simulink model "Control_Schematic_13a"  (Simulink 8.3)
settings: Solver=ode3  StartTime=0.0  StopTime=350  FixedStep=Ts  RelTol=1e-3
values from neighbouring files (symbols this model uses):
  b = 156    [StartUp_1.m]    (also in StartUp_11_Validation.m; StartUp_3.m; StartUp_4.m; StartUp_7.m)
  Eps = .1    (= 0.1)    [StartUp_9.m]
  K1 = PolyCon(1,2)    [StartUp_1.m]    (also in StartUp_4.m = 1; StartUp_7.m = 16; StartUp_8.m = 16; StartUp_9.m = 0.23)
  k2 = floor(rk(2,1))    [StartUp_9.m]
  K2 = 2    [StartUp_4.m]    (also in StartUp_7.m = 8; StartUp_8.m = 8; StartUp_9.m = 0.83)
  K3 = 12000    [StartUp_9.m]
  Kn = .0019    (= 0.0019)    [StartUp_9.m]
  r = 820    [StartUp_1.m]    (also in StartUp_11_Validation.m = 50; StartUp_3.m = 520; StartUp_4.m = 0.01; StartUp_7.m = 0.01)
  TD = ss(Atd,Btd,Ctd,Dtd,Ts)    [StartUp_1.m]    (also in StartUp_3.m; StartUp_4.m; StartUp_7.m; StartUp_8.m)
  Ts = 1/1000    (= 0.001)    [StartUp_1.m]    (also in StartUp_11_Validation.m = 0.01; StartUp_3.m; StartUp_4.m; StartUp_7.m)
  x_0 = 2500    [StartUp_9.m]
  y_0 = 2500    [StartUp_9.m]
undefined symbols (not defined in the file or in its folder): d0t, DiscIntNeverNeededParam, dt, ht, k1, rho1, rho2, rt
libraries: simulink x2, dspinverses x1
settings Model: Creator=baqumau  LastModifiedBy=baqumau
settings DataIOCC: SignalLoggingSaveFormat=Dataset
settings DebuggingCC: UnderspecifiedInitializationDetection=Simplified  StateNameClashWarn=none
settings GRTTargetCC: CombineOutputUpdateFcns=on  GRTInterface=off

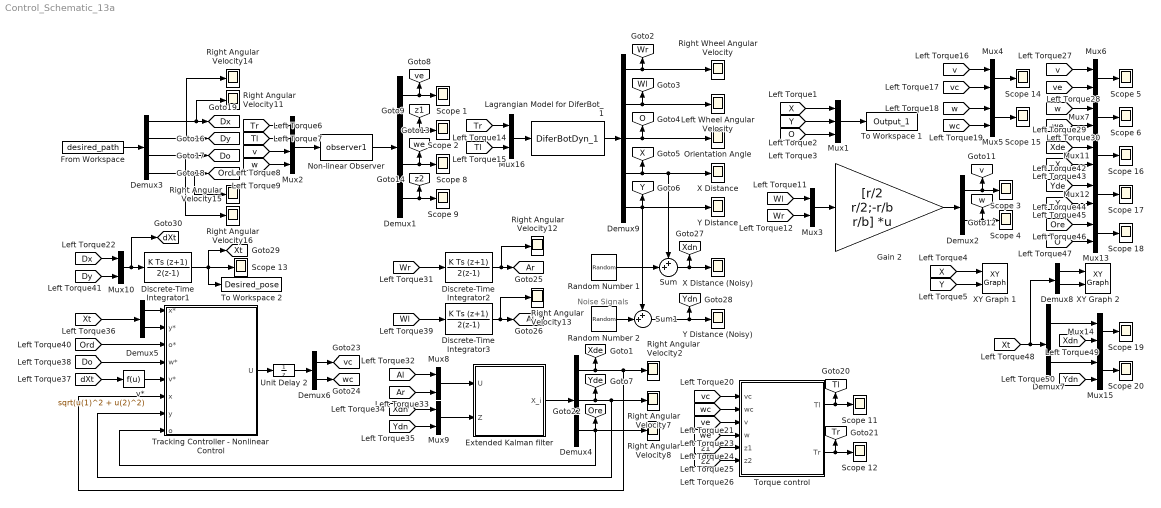
== system Control_Schematic_13a ==
  note: Noise Signals
  Demux1 : Demux
  Demux{2,5..8} (5 alike) : Demux  Outputs=2
  Demux3 : Demux
  Demux4 : Demux  Outputs=3
  Demux9 : Demux  Outputs=5
  Discrete-Time Integrator1 : DiscreteIntegrator  IntegratorMethod=Integration: Trapezoidal  gainval=1  InitialCondition=[x_0,y_0]'  SampleTime=Ts  ICPrevOutput=DiscIntNeverNeededParam  ICPrevScaledInput=DiscIntNeverNeededParam
  Discrete-Time Integrator2 : DiscreteIntegrator  IntegratorMethod=Integration: Trapezoidal  gainval=1  SampleTime=Ts  ICPrevOutput=DiscIntNeverNeededParam  ICPrevScaledInput=DiscIntNeverNeededParam
  Discrete-Time Integrator3 : DiscreteIntegrator  IntegratorMethod=Integration: Trapezoidal  gainval=1  SampleTime=Ts  ICPrevOutput=DiscIntNeverNeededParam  ICPrevScaledInput=DiscIntNeverNeededParam
  Extended Kalman filter : Subsystem
  From Workspace : FromWorkspace  VariableName=desired_path  SampleTime=Ts  OutputAfterFinalValue=Holding final value
  Gain 2 : Gain  Gain=[r/2 r/2;-r/b r/b]  Multiplication=Matrix(K*u)
  Lagrangian Model for DiferBot_1 : S-Function  FunctionName=DiferBotDyn_1  Parameters=par  EnableBusSupport=off
  Left Wheel Angular Velocity : Scope
      settings: YMin=-1  YMax=1  SaveName=ScopeData2
  Mux1 : Mux  Inputs=3
  Mux{3..16} (14 alike) : Mux  Inputs=2
  Mux2 : Mux
  Non-linear Observer : S-Function  FunctionName=observer1  Parameters=par  EnableBusSupport=off
  Orientation Angle : Scope
      settings: YMin=-3  YMax=3
  Random Number 1 : RandomNumber  Variance=.5  Seed=6  SampleTime=Ts
  Random Number 2 : RandomNumber  Variance=.5  Seed=8  SampleTime=Ts
  Right Angular Velocity{2,7..8,11..16} (9 alike) : Scope
      Right Angular Velocity11 settings: YMin=0  YMax=4500  SaveName=ScopeData17
      Right Angular Velocity12 settings: YMin=-3  YMax=30  SaveName=ScopeData39
      Right Angular Velocity13 settings: YMin=-3  YMax=3  SaveName=ScopeData40
      Right Angular Velocity14 settings: TimeRange=500  YMin=0  YMax=4500  SaveName=ScopeData20
      Right Angular Velocity15 settings: YMin=-3.141592653589793  YMax=3.141592653589793  SaveName=ScopeData15
      Right Angular Velocity16 settings: YMin=-0.1  YMax=-0.1  SaveName=ScopeData16
      Right Angular Velocity2 settings: YMin=2400  YMax=2600  SaveName=ScopeData35
      Right Angular Velocity7 settings: YMin=0  YMax=5000  SaveName=ScopeData36
      Right Angular Velocity8 settings: YMin=-3.141592653589793  YMax=3.141592653589793  SaveName=ScopeData37
  Right Wheel Angular Velocity : Scope
      settings: YMin=-1  YMax=20  SaveName=ScopeData3
  Scope {1..6,8..9,11..20} (18 alike) : Scope
      Scope 1 settings: YMin=0  YMax=5000  SaveName=ScopeData5
      Scope 11 settings: YMin=-20  YMax=20  SaveName=ScopeData24
      Scope 12 settings: YMin=-15  YMax=15  SaveName=ScopeData25
      Scope 13 settings: YMin=100  YMax=5000  SaveName=ScopeData42
      Scope 14 settings: YMin=-150  YMax=150  SaveName=ScopeData18
      Scope 15 settings: YMin=-2  YMax=2  SaveName=ScopeData19
      Scope 16 settings: YMin=0  YMax=5000  SaveName=ScopeData43
      Scope 17 settings: YMin=0  YMax=10000  SaveName=ScopeData46
      Scope 18 settings: YMin=-10  YMax=1.1  SaveName=ScopeData51
      Scope 19 settings: YMin=0  YMax=5000  SaveName=ScopeData52
      Scope 2 settings: YMin=-100  YMax=200  SaveName=ScopeData6
      Scope 20 settings: YMin=0  YMax=5000  SaveName=ScopeData53
      Scope 3 settings: YMin=0  YMax=5000  SaveName=ScopeData10
      Scope 4 settings: YMin=0  YMax=5000  SaveName=ScopeData11
      Scope 5 settings: YMin=-150  YMax=500  SaveName=ScopeData28
      Scope 6 settings: SaveName=ScopeData29
      Scope 8 settings: YMin=-1  YMax=1  SaveName=ScopeData12
      Scope 9 settings: TimeRange=388  YMin=-6  YMax=6  SaveName=ScopeData14
  Sum : Sum  Inputs=++|
  Sum1 : Sum  Inputs=++|
  To Workspace 1 : ToWorkspace  VariableName=Output_1  SaveFormat=Structure With Time  SampleTime=-1
  To Workspace 2 : ToWorkspace  VariableName=Desired_pose  SaveFormat=Structure With Time  SampleTime=-1
  Torque control : Subsystem
  Tracking Controller - Nonlinear Control : Subsystem
  Unit Delay 2 : UnitDelay  SampleTime=-1
  X Distance : Scope
      settings: YMin=0  YMax=5000  SaveName=ScopeData4
  X Distance (Noisy) : Scope
      settings: YMin=0  YMax=2600  SaveName=ScopeData38
  XY Graph 1 : simulink/Sinks/XY Graph  xmin=0  xmax=5000  ymin=0  ymax=5000  st=-1
  XY Graph 2 : simulink/Sinks/XY Graph  xmin=0  xmax=5000  ymin=0  ymax=5000  st=-1
  Y Distance : Scope
      settings: YMin=0  YMax=5000
  Y Distance (Noisy) : Scope
      settings: YMin=0  YMax=2600  SaveName=ScopeData41
  v* : Fcn  Expr=sqrt(u(1)^2 + u(2)^2)
  tag scope: Al=global, Ar=global, Do=global, Dx=global, Dy=global, O=global, Ord=global, Ore=global, Tl=global, Tr=global, Wl=global, Wr=global, X=global, Xde=global, Xdn=global, Xt=global, Y=global, Yde=global, Ydn=global, dXt=global, v=global, vc=global, ve=global, w=global, wc=global, we=global, z1=global, z2=global
  wires:
  Demux9/1 -> Right Wheel Angular Velocity/1, [Wr]
  Demux9/2 -> Left Wheel Angular Velocity/1, [Wl]
  Demux9/3 -> Orientation Angle/1, [O]
  [X] -> Mux1/1
  [Y] -> Mux1/2
  [O] -> Mux1/3
  Mux1/1 -> To Workspace 1/1
  [X] -> XY Graph 1/1
  [Y] -> XY Graph 1/2
  [Wl] -> Mux3/1
  [Wr] -> Mux3/2
  Mux3/1 -> Gain 2/1
  Gain 2/1 -> Demux2/1
  Demux2/2 -> Scope 4/1, [w]
  Demux2/1 -> Scope 3/1, [v]
  Mux2/1 -> Non-linear Observer/1
  [Tr] -> Mux2/1
  [Tl] -> Mux2/2
  [v] -> Mux2/3
  [w] -> Mux2/4
  Non-linear Observer/1 -> Demux1/1
  Demux1/2 -> [z1], Scope 2/1
  Demux1/1 -> [ve], Scope 1/1
  Demux1/4 -> [z2], Scope 9/1
  [vc] -> Mux4/2
  [v] -> Mux4/1
  Mux4/1 -> Scope 14/1
  [wc] -> Mux5/2
  [w] -> Mux5/1
  Mux5/1 -> Scope 15/1
  Demux3/1 -> Right Angular Velocity11/1, [Dx]
  Demux3/2 -> Right Angular Velocity14/1, [Dy]
  Demux3/3 -> Right Angular Velocity16/1, [Do]
  Demux3/4 -> Right Angular Velocity15/1, [Ord]
  From Workspace/1 -> Demux3/1
  [vc] -> Torque control/1(vc)
  [wc] -> Torque control/2(wc)
  [ve] -> Torque control/3(v)
  [we] -> Torque control/4(w)
  [z1] -> Torque control/5(z1)
  [z2] -> Torque control/6(z2)
  Torque control/2(Tr) -> [Tr], Scope 12/1
  Torque control/1(Tl) -> [Tl], Scope 11/1
  [Tr] -> Mux16/1
  [ve] -> Mux6/2
  [v] -> Mux6/1
  Mux6/1 -> Scope 5/1
  [we] -> Mux7/2
  [w] -> Mux7/1
  Mux7/1 -> Scope 6/1
  [Ar] -> Mux8/2
  [Al] -> Mux8/1
  [Ydn] -> Mux9/2
  [Xdn] -> Mux9/1
  Mux8/1 -> Extended Kalman filter/1(U)
  Mux9/1 -> Extended Kalman filter/2(Z)
  Demux4/2 -> [Yde], Tracking Controller - Nonlinear Control/7(y), Right Angular Velocity7/1
  Demux4/3 -> Tracking Controller - Nonlinear Control/8(o), [Ore], Right Angular Velocity8/1
  Demux4/1 -> [Xde], Tracking Controller - Nonlinear Control/6(x), Right Angular Velocity2/1
  Demux6/2 -> [wc]
  Demux6/1 -> [vc]
  Discrete-Time Integrator2/1 -> Right Angular Velocity12/1, [Ar]
  [Wr] -> Discrete-Time Integrator2/1
  Discrete-Time Integrator3/1 -> Right Angular Velocity13/1, [Al]
  [Wl] -> Discrete-Time Integrator3/1
  Tracking Controller - Nonlinear Control/1(U) -> Unit Delay 2/1
  Demux5/1 -> Tracking Controller - Nonlinear Control/1(x*)
  Demux5/2 -> Tracking Controller - Nonlinear Control/2(y*)
  [Xt] -> Demux5/1
  [Do] -> Tracking Controller - Nonlinear Control/4(w*)
  v*/1 -> Tracking Controller - Nonlinear Control/5(v*)
  [dXt] -> v*/1
  [Ord] -> Tracking Controller - Nonlinear Control/3(o*)
  Extended Kalman filter/1(X_i) -> Demux4/1
  Unit Delay 2/1 -> Demux6/1
  Demux9/4 -> X Distance/1, Sum/1, [X]
  Demux9/5 -> Y Distance/1, Sum1/1, [Y]
  Random Number 1/1 -> Sum/2
  Sum1/1 -> Y Distance (Noisy)/1, [Ydn]
  Sum/1 -> [Xdn], X Distance (Noisy)/1
  Random Number 2/1 -> Sum1/2
  Discrete-Time Integrator1/1 -> [Xt], To Workspace 2/1, Scope 13/1
  [Dx] -> Mux10/1
  [Dy] -> Mux10/2
  Mux10/1 -> [dXt], Discrete-Time Integrator1/1
  [X] -> Mux11/2
  [Xde] -> Mux11/1
  Mux11/1 -> Scope 16/1
  [Y] -> Mux12/2
  [Yde] -> Mux12/1
  Mux12/1 -> Scope 17/1
  [O] -> Mux13/2
  [Ore] -> Mux13/1
  Mux13/1 -> Scope 18/1
  [Xt] -> Demux8/1, Demux7/1
  Demux7/1 -> Mux14/1
  [Xdn] -> Mux14/2
  Demux7/2 -> Mux15/1
  [Ydn] -> Mux15/2
  Mux14/1 -> Scope 19/1
  Mux15/1 -> Scope 20/1
  Demux1/3 -> [we], Scope 8/1
  Demux8/2 -> XY Graph 2/2
  Demux8/1 -> XY Graph 2/1
  Lagrangian Model for DiferBot_1/1 -> Demux9/1
  Mux16/1 -> Lagrangian Model for DiferBot_1/1
  [Tl] -> Mux16/2

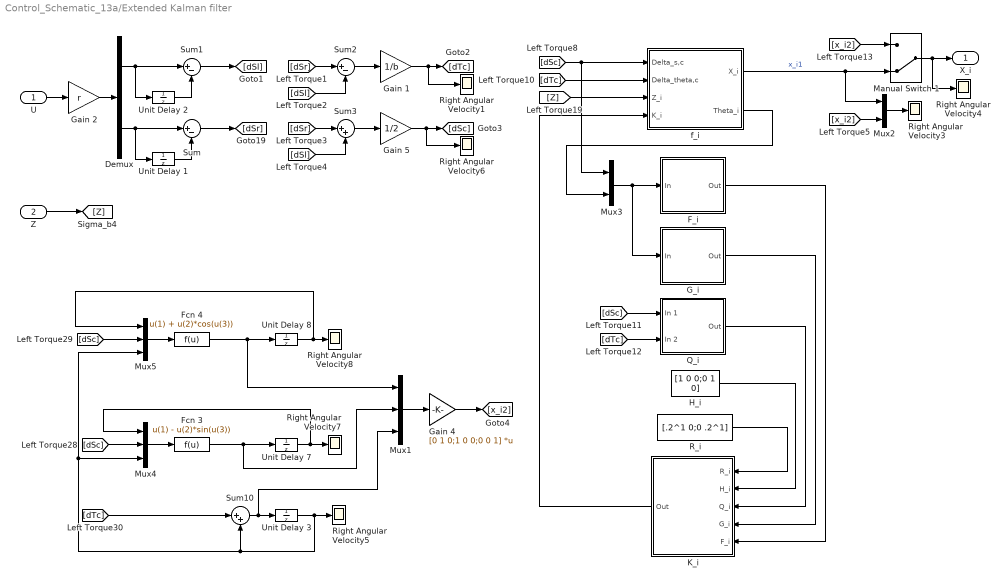
== system Control_Schematic_13a/Extended Kalman filter ==
  U : Inport
  Z : Inport  Port=2
  Demux : Demux  Outputs=2
  F_i : Subsystem
  Fcn 3 : Fcn  Expr=u(1) - u(2)*sin(u(3))
  Fcn 4 : Fcn  Expr=u(1) + u(2)*cos(u(3))
  G_i : Subsystem
  Gain 1 : Gain  Gain=1/b
  Gain 2 : Gain  Gain=r
  Gain 4 : Gain  Gain=[0 1 0;1 0 0;0 0 1]  Multiplication=Matrix(K*u)
  Gain 5 : Gain  Gain=1/2
  H_i : Constant  Value=[1 0 0;0 1 0]
  K_i : Subsystem
  Manual Switch 1 : ManualSwitch  CurrentSetting=0
  Mux1 : Mux  Inputs=3
  Mux2 : Mux  Inputs=2
  Mux3 : Mux  Inputs=2
  Mux4 : Mux  Inputs=3
  Mux5 : Mux  Inputs=3
  Q_i : Subsystem
  R_i : Constant  Value=[.2^1 0;0 .2^1]
  Right Angular Velocity{1,3..8} (7 alike) : Scope
      Right Angular Velocity1 settings: YMin=-1  YMax=1  SaveName=ScopeData23
      Right Angular Velocity3 settings: YMin=-1  YMax=2  SaveName=ScopeData29
      Right Angular Velocity4 settings: YMin=-1  YMax=1  SaveName=ScopeData31
      Right Angular Velocity5 settings: YMin=-1  YMax=3  SaveName=ScopeData32
      Right Angular Velocity6 settings: YMin=-1  YMax=1  SaveName=ScopeData22
      Right Angular Velocity7 settings: YMin=2490  YMax=2510  SaveName=ScopeData33
      Right Angular Velocity8 settings: YMin=100  YMax=500  SaveName=ScopeData34
  Sum : Sum  Inputs=|+-
  Sum1 : Sum  Inputs=|+-
  Sum10 : Sum  Inputs=|++
  Sum2 : Sum  Inputs=|+-
  Sum3 : Sum  Inputs=|++
  Unit Delay 1 : UnitDelay  SampleTime=-1
  Unit Delay 2 : UnitDelay  SampleTime=-1
  Unit Delay 3 : UnitDelay  SampleTime=-1
  Unit Delay 7 : UnitDelay  InitialCondition=2500  SampleTime=-1
  Unit Delay 8 : UnitDelay  InitialCondition=200  SampleTime=-1
  f_i : Subsystem
  X_i : Outport
  wires:
  U/1 -> Gain 2/1
  Demux/2 -> Unit Delay 1/1, Sum/1
  Unit Delay 1/1 -> Sum/2
  Sum/1 -> [dSr]
  Demux/1 -> Sum1/1, Unit Delay 2/1
  Unit Delay 2/1 -> Sum1/2
  Sum1/1 -> [dSl]
  [dSr] -> Sum2/1
  [dSl] -> Sum2/2
  Sum2/1 -> Gain 1/1
  Gain 1/1 -> Right Angular Velocity1/1, [dTc]
  [dSr] -> Sum3/1
  [dSl] -> Sum3/2
  Sum3/1 -> Gain 5/1
  Gain 5/1 -> Right Angular Velocity6/1, [dSc]
  [dSc] -> Mux3/1, f_i/1(Delta_s,c)
  Mux3/1 -> G_i/1(In), F_i/1(In)
  Sum10/1 -> Mux1/3, Unit Delay 3/1
  Unit Delay 3/1 -> Right Angular Velocity5/1, Mux5/3, Mux4/3, Sum10/2
  Unit Delay 7/1 -> Mux4/1, Right Angular Velocity7/1
  Fcn 3/1 -> Mux1/2, Unit Delay 7/1
  [dSc] -> Mux4/2
  Mux4/1 -> Fcn 3/1
  Fcn 4/1 -> Mux1/1, Unit Delay 8/1
  Mux5/1 -> Fcn 4/1
  Unit Delay 8/1 -> Mux5/1, Right Angular Velocity8/1
  [dSc] -> Mux5/2
  Gain 2/1 -> Demux/1
  Z/1 -> [Z]
  [Z] -> f_i/3(Z_i)
  [dTc] -> f_i/2(Delta_theta,c)
  [dSc] -> Q_i/1(In 1)
  [dTc] -> Q_i/2(In 2)
  Mux1/1 -> Gain 4/1
  Gain 4/1 -> [x_i2]
  Manual Switch 1/1 -> Right Angular Velocity4/1, X_i/1
  [x_i2] -> Manual Switch 1/1
  f_i/1(X_i) -> Mux2/1, Manual Switch 1/2  "x_i1"
  [x_i2] -> Mux2/2
  Mux2/1 -> Right Angular Velocity3/1
  [dTc] -> Sum10/1
  K_i/1(Out) -> f_i/4(K_i)
  f_i/2(Theta_i) -> Mux3/2
  F_i/1(Out) -> K_i/5(F_i)
  G_i/1(Out) -> K_i/4(G_i)
  Q_i/1(Out) -> K_i/3(Q_i)
  H_i/1 -> K_i/2(H_i)
  R_i/1 -> K_i/1(R_i)

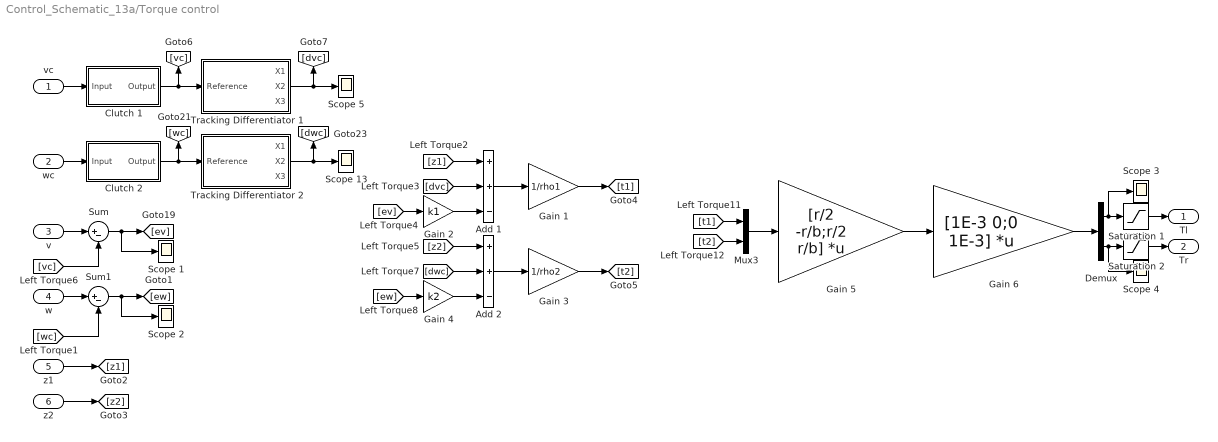
== system Control_Schematic_13a/Torque control ==
  vc : Inport
  wc : Inport  Port=2
  v : Inport  Port=3
  w : Inport  Port=4
  z1 : Inport  Port=5
  z2 : Inport  Port=6
  Add 1 : Sum  Inputs=++-
  Add 2 : Sum  Inputs=++-
  Clutch 1 : Subsystem
  Clutch 2 : Subsystem
  Demux : Demux  Outputs=2
  Gain 1 : Gain  Gain=1/rho1
  Gain 2 : Gain  Gain=k1
  Gain 3 : Gain  Gain=1/rho2
  Gain 4 : Gain  Gain=k2
  Gain 5 : Gain  Gain=[r/2 -r/b;r/2 r/b]  Multiplication=Matrix(K*u)
  Gain 6 : Gain  Gain=[1E-3 0;0 1E-3]  Multiplication=Matrix(K*u)
  Mux3 : Mux  Inputs=2
  Saturation 1 : Saturate  UpperLimit=15  LowerLimit=-15
  Saturation 2 : Saturate  UpperLimit=15  LowerLimit=-15
  Scope {1..5,13} (6 alike) : Scope
      Scope 1 settings: YMin=-500  YMax=500  SaveName=ScopeData7
      Scope 13 settings: YMin=0  YMax=5000  SaveName=ScopeData23
      Scope 2 settings: YMin=-10  YMax=10  SaveName=ScopeData8
      Scope 3 settings: YMin=0  YMax=5000  SaveName=ScopeData26
      Scope 4 settings: YMin=0  YMax=5000  SaveName=ScopeData27
      Scope 5 settings: YMin=0  YMax=5000  SaveName=ScopeData21
  Sum : Sum  Inputs=|+-
  Sum1 : Sum  Inputs=|+-
  Tracking Differentiator 1 : Subsystem
  Tracking Differentiator 2 : Subsystem
  Tl : Outport
  Tr : Outport  Port=2
  wires:
  wc/1 -> Clutch 2/1(Input)
  Tracking Differentiator 2/2(X2) -> Scope 13/1, [dwc]
  v/1 -> Sum/1
  [vc] -> Sum/2
  Sum/1 -> Scope 1/1, [ev]
  w/1 -> Sum1/1
  [wc] -> Sum1/2
  Sum1/1 -> Scope 2/1, [ew]
  z1/1 -> [z1]
  z2/1 -> [z2]
  Add 1/1 -> Gain 1/1
  Gain 1/1 -> [t1]
  [z1] -> Add 1/1
  [dvc] -> Add 1/2
  Gain 2/1 -> Add 1/3
  [ev] -> Gain 2/1
  Add 2/1 -> Gain 3/1
  Gain 3/1 -> [t2]
  [z2] -> Add 2/1
  [dwc] -> Add 2/2
  Gain 4/1 -> Add 2/3
  [ew] -> Gain 4/1
  [t1] -> Mux3/1
  [t2] -> Mux3/2
  Mux3/1 -> Gain 5/1
  Gain 5/1 -> Gain 6/1
  Demux/1 -> Scope 3/1, Saturation 1/1
  Demux/2 -> Scope 4/1, Saturation 2/1
  Saturation 1/1 -> Tl/1
  Saturation 2/1 -> Tr/1
  Gain 6/1 -> Demux/1
  vc/1 -> Clutch 1/1(Input)
  Tracking Differentiator 1/2(X2) -> Scope 5/1, [dvc]
  Clutch 1/1(Output) -> Tracking Differentiator 1/1(Reference), [vc]
  Clutch 2/1(Output) -> Tracking Differentiator 2/1(Reference), [wc]

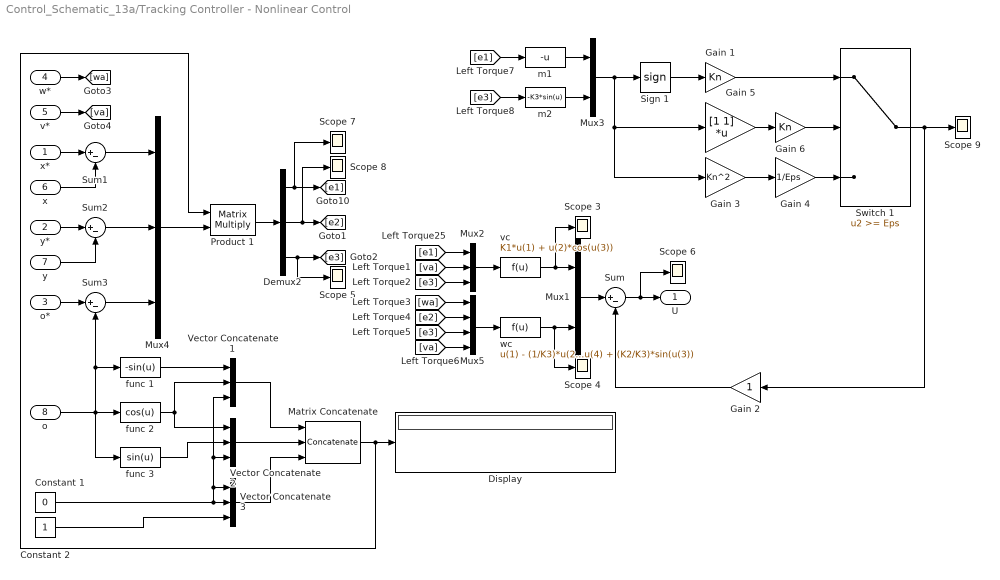
== system Control_Schematic_13a/Tracking Controller - Nonlinear Control ==
  x* : Inport
  y* : Inport  Port=2
  o* : Inport  Port=3
  w* : Inport  Port=4
  v* : Inport  Port=5
  x : Inport  Port=6
  y : Inport  Port=7
  o : Inport  Port=8
  Constant 1 : Constant  Value=0
  Constant 2 : Constant
  Demux2 : Demux  Outputs=3
  Display : Display
  Gain 1 : Gain  Gain=Kn
  Gain 2 : Gain
  Gain 3 : Gain  Gain=Kn^2
  Gain 4 : Gain  Gain=1/Eps
  Gain 5 : Gain  Gain=[1 1]  Multiplication=Matrix(K*u)
  Gain 6 : Gain  Gain=Kn
  Matrix Concatenate : Concatenate  NumInputs=3  Mode=Multidimensional array  ConcatenateDimension=2
  Mux1 : Mux  Inputs=2
  Mux2 : Mux  Inputs=3
  Mux3 : Mux  Inputs=2
  Mux4 : Mux  Inputs=3
  Mux5 : Mux
  Product 1 : Product  Multiplication=Matrix(*)
  Scope {3..9} (7 alike) : Scope
      Scope 3 settings: YMin=-10  YMax=10  SaveName=ScopeData44
      Scope 4 settings: YMin=-400  YMax=1300  SaveName=ScopeData45
      Scope 5 settings: SaveName=ScopeData47
      Scope 6 settings: TimeRange=388.54  YMin=-0.5  YMax=0.5  SaveName=ScopeData12
      Scope 7 settings: YMin=-10  YMax=10  SaveName=ScopeData48
      Scope 8 settings: YMin=-10  YMax=10  SaveName=ScopeData49
      Scope 9 settings: YMin=-0.1  YMax=0.1  SaveName=ScopeData50
  Sign 1 : Signum
  Sum{,1..3} (4 alike) : Sum  Inputs=|+-
  Switch 1 : Switch  Threshold=Eps
  Vector Concatenate 1 : Concatenate  NumInputs=3
  Vector Concatenate 2 : Concatenate  NumInputs=3
  Vector Concatenate 3 : Concatenate  NumInputs=3
  func 1 : Fcn  Expr=-sin(u)
  func 2 : Fcn  Expr=cos(u)
  func 3 : Fcn  Expr=sin(u)
  m1 : Fcn  Expr=-u
  m2 : Fcn  Expr=-K3*sin(u)
  vc : Fcn  Expr=K1*u(1) + u(2)*cos(u(3))
  wc : Fcn  Expr=u(1) - (1/K3)*u(2)*u(4) + (K2/K3)*sin(u(3))
  U : Outport
  wires:
  Sum/1 -> Scope 6/1, U/1
  wc/1 -> Scope 4/1, Mux1/2
  vc/1 -> Scope 3/1, Mux1/1
  m2/1 -> Mux3/2
  m1/1 -> Mux3/1
  Mux3/1 -> Gain 5/1, Gain 3/1, Sign 1/1
  Sign 1/1 -> Gain 1/1
  Mux1/1 -> Sum/1
  func 2/1 -> Vector Concatenate 1/2, Vector Concatenate 2/1
  func 3/1 -> Vector Concatenate 2/2
  func 1/1 -> Vector Concatenate 1/1
  o/1 -> func 3/1, func 2/1, Sum3/2, func 1/1
  Constant 1/1 -> Vector Concatenate 3/1, Vector Concatenate 2/3, Vector Concatenate 1/3, Vector Concatenate 3/2
  Constant 2/1 -> Vector Concatenate 3/3
  Matrix Concatenate/1 -> Product 1/1, Display/1
  Vector Concatenate 1/1 -> Matrix Concatenate/1
  Vector Concatenate 2/1 -> Matrix Concatenate/2
  Vector Concatenate 3/1 -> Matrix Concatenate/3
  x*/1 -> Sum1/1
  x/1 -> Sum1/2
  y*/1 -> Sum2/1
  y/1 -> Sum2/2
  o*/1 -> Sum3/1
  Sum3/1 -> Mux4/3
  Sum1/1 -> Mux4/1
  Sum2/1 -> Mux4/2
  Mux4/1 -> Product 1/2
  Product 1/1 -> Demux2/1
  Demux2/1 -> Scope 7/1, [e1]
  Demux2/2 -> Scope 8/1, [e2]
  Demux2/3 -> Scope 5/1, [e3]
  [e1] -> Mux2/1
  w*/1 -> [wa]
  v*/1 -> [va]
  [va] -> Mux2/2
  [e3] -> Mux2/3
  Mux2/1 -> vc/1
  Mux5/1 -> wc/1
  [wa] -> Mux5/1
  [e2] -> Mux5/2
  [e3] -> Mux5/3
  [va] -> Mux5/4
  [e1] -> m1/1
  [e3] -> m2/1
  Gain 2/1 -> Sum/2
  Gain 3/1 -> Gain 4/1
  Gain 5/1 -> Gain 6/1
  Gain 4/1 -> Switch 1/3
  Gain 6/1 -> Switch 1/2
  Gain 1/1 -> Switch 1/1
  Switch 1/1 -> Scope 9/1, Gain 2/1

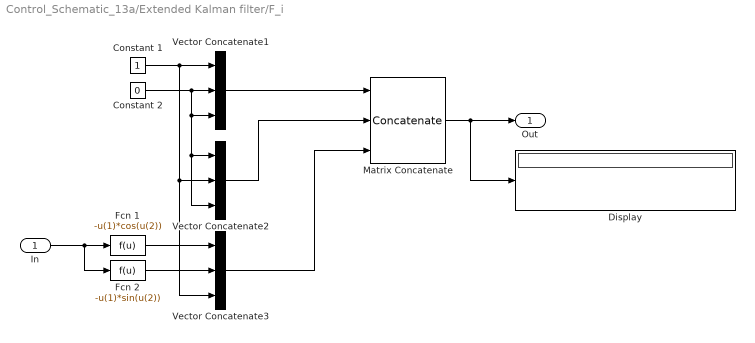
== system Control_Schematic_13a/Extended Kalman filter/F_i ==
  In : Inport
  Constant 1 : Constant
  Constant 2 : Constant  Value=0
  Display : Display
  Fcn 1 : Fcn  Expr=-u(1)*cos(u(2))
  Fcn 2 : Fcn  Expr=-u(1)*sin(u(2))
  Matrix Concatenate : Concatenate  NumInputs=3  Mode=Multidimensional array  ConcatenateDimension=2
  Vector Concatenate1 : Concatenate  NumInputs=3
  Vector Concatenate2 : Concatenate  NumInputs=3
  Vector Concatenate3 : Concatenate  NumInputs=3
  Out : Outport
  wires:
  In/1 -> Fcn 2/1, Fcn 1/1
  Matrix Concatenate/1 -> Display/1, Out/1
  Constant 1/1 -> Vector Concatenate3/3, Vector Concatenate2/2, Vector Concatenate1/1
  Constant 2/1 -> Vector Concatenate2/3, Vector Concatenate2/1, Vector Concatenate1/3, Vector Concatenate1/2
  Vector Concatenate1/1 -> Matrix Concatenate/1
  Vector Concatenate2/1 -> Matrix Concatenate/2
  Fcn 1/1 -> Vector Concatenate3/1
  Fcn 2/1 -> Vector Concatenate3/2
  Vector Concatenate3/1 -> Matrix Concatenate/3

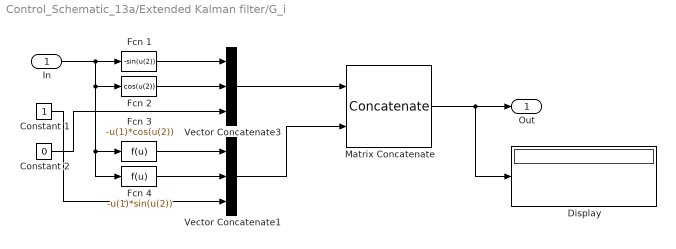
== system Control_Schematic_13a/Extended Kalman filter/G_i ==
  In : Inport
  Constant 1 : Constant
  Constant 2 : Constant  Value=0
  Display : Display
  Fcn 1 : Fcn  Expr=-sin(u(2))
  Fcn 2 : Fcn  Expr=cos(u(2))
  Fcn 3 : Fcn  Expr=-u(1)*cos(u(2))
  Fcn 4 : Fcn  Expr=-u(1)*sin(u(2))
  Matrix Concatenate : Concatenate  Mode=Multidimensional array  ConcatenateDimension=2
  Vector Concatenate1 : Concatenate  NumInputs=3
  Vector Concatenate3 : Concatenate  NumInputs=3
  Out : Outport
  wires:
  Fcn 2/1 -> Vector Concatenate3/2
  Fcn 1/1 -> Vector Concatenate3/1
  Matrix Concatenate/1 -> Display/1, Out/1
  In/1 -> Fcn 1/1, Fcn 2/1, Fcn 4/1, Fcn 3/1
  Vector Concatenate3/1 -> Matrix Concatenate/1
  Vector Concatenate1/1 -> Matrix Concatenate/2
  Constant 2/1 -> Vector Concatenate3/3
  Constant 1/1 -> Vector Concatenate1/3
  Fcn 3/1 -> Vector Concatenate1/1
  Fcn 4/1 -> Vector Concatenate1/2

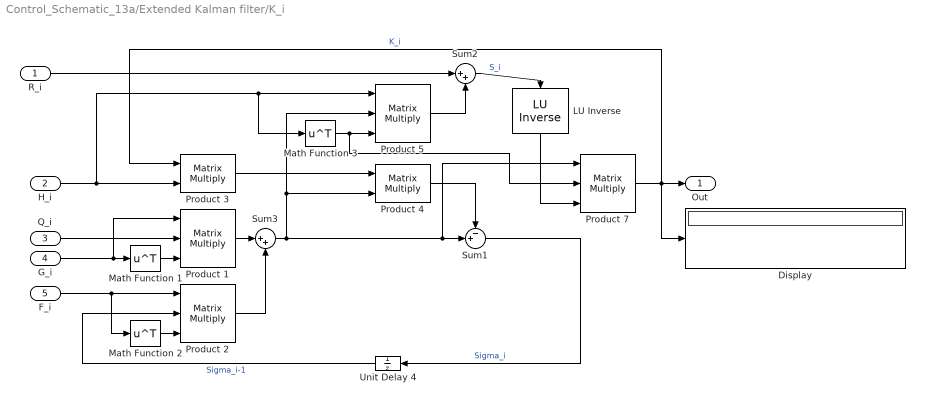
== system Control_Schematic_13a/Extended Kalman filter/K_i ==
  R_i : Inport
  H_i : Inport  Port=2
  Q_i : Inport  Port=3
  G_i : Inport  Port=4
  F_i : Inport  Port=5
  " LU Inverse" : dspinverses/ LU Inverse
  Display : Display
  Math Function 1 : Math  Operator=transpose  SaturateOnIntegerOverflow=on
  Math Function 2 : Math  Operator=transpose  SaturateOnIntegerOverflow=on
  Math Function 3 : Math  Operator=transpose  SaturateOnIntegerOverflow=on
  Product {1..2,5,7} (4 alike) : Product  Inputs=3  Multiplication=Matrix(*)
  Product 3 : Product  Multiplication=Matrix(*)
  Product 4 : Product  Multiplication=Matrix(*)
  Sum1 : Sum  Inputs=-+|
  Sum2 : Sum  Inputs=|++
  Sum3 : Sum  Inputs=|++
  Unit Delay 4 : UnitDelay  InitialCondition=[1 0 0;0 1 0;0 0 1]  SampleTime=-1
  Out : Outport
  wires:
  Q_i/1 -> Product 1/2
  G_i/1 -> Math Function 1/1, Product 1/1
  Math Function 1/1 -> Product 1/3
  F_i/1 -> Math Function 2/1, Product 2/1
  Unit Delay 4/1 -> Product 2/2  "Sigma_i-1"
  Math Function 2/1 -> Product 2/3
  Product 1/1 -> Sum3/1
  Product 2/1 -> Sum3/2
  H_i/1 -> Product 5/1, Math Function 3/1, Product 3/2
  Product 7/1 -> Out/1, Display/1, Product 3/1  "K_i"
  Product 3/1 -> Product 4/1
  Sum3/1 -> Product 7/1, Sum1/2, Product 4/2, Product 5/2
  Product 4/1 -> Sum1/1
  Sum1/1 -> Unit Delay 4/1  "Sigma_i"
  Math Function 3/1 -> Product 5/3, Product 7/2
  R_i/1 -> Sum2/1
  Product 5/1 -> Sum2/2
  Sum2/1 -> " LU Inverse"/1  "S_i"
  " LU Inverse"/1 -> Product 7/3

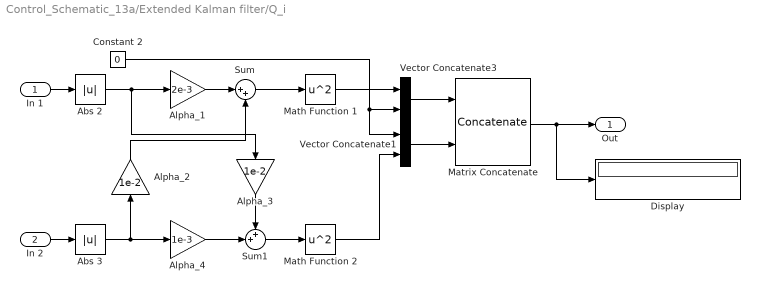
== system Control_Schematic_13a/Extended Kalman filter/Q_i ==
  In 1 : Inport
  In 2 : Inport  Port=2
  Abs 2 : Abs
  Abs 3 : Abs
  Alpha_1 : Gain  Gain=2e-3
  Alpha_2 : Gain  Gain=1e-2
  Alpha_3 : Gain  Gain=1e-2
  Alpha_4 : Gain  Gain=1e-3
  Constant 2 : Constant  Value=0
  Display : Display
  Math Function 1 : Math  Operator=square  SaturateOnIntegerOverflow=on
  Math Function 2 : Math  Operator=square  SaturateOnIntegerOverflow=on
  Matrix Concatenate : Concatenate  Mode=Multidimensional array  ConcatenateDimension=2
  Sum : Sum  Inputs=|++
  Sum1 : Sum  Inputs=++|
  Vector Concatenate1 : Concatenate
  Vector Concatenate3 : Concatenate
  Out : Outport
  wires:
  Vector Concatenate1/1 -> Matrix Concatenate/2
  Vector Concatenate3/1 -> Matrix Concatenate/1
  Matrix Concatenate/1 -> Display/1, Out/1
  In 1/1 -> Abs 2/1
  In 2/1 -> Abs 3/1
  Abs 2/1 -> Alpha_3/1, Alpha_1/1
  Abs 3/1 -> Alpha_4/1, Alpha_2/1
  Constant 2/1 -> Vector Concatenate3/2, Vector Concatenate1/1
  Alpha_1/1 -> Sum/1
  Alpha_2/1 -> Sum/2
  Sum/1 -> Math Function 1/1
  Math Function 1/1 -> Vector Concatenate3/1
  Alpha_4/1 -> Sum1/2
  Alpha_3/1 -> Sum1/1
  Sum1/1 -> Math Function 2/1
  Math Function 2/1 -> Vector Concatenate1/2

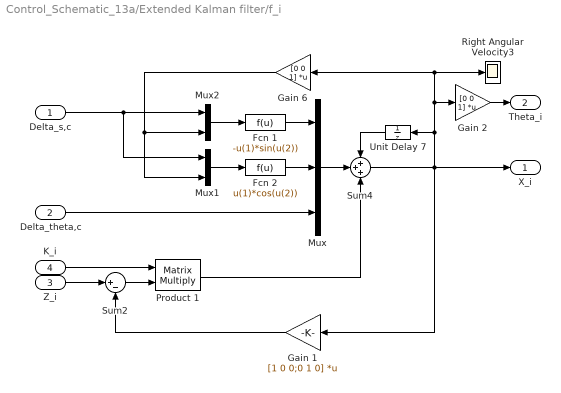
== system Control_Schematic_13a/Extended Kalman filter/f_i ==
  Delta_s,c : Inport
  Delta_theta,c : Inport  Port=2
  Z_i : Inport  Port=3
  K_i : Inport  Port=4
  Fcn 1 : Fcn  Expr=-u(1)*sin(u(2))
  Fcn 2 : Fcn  Expr=u(1)*cos(u(2))
  Gain 1 : Gain  Gain=[1 0 0;0 1 0]  Multiplication=Matrix(K*u)
  Gain 2 : Gain  Gain=[0 0 1]  Multiplication=Matrix(K*u)
  Gain 6 : Gain  Gain=[0 0 1]  Multiplication=Matrix(K*u)
  Mux : Mux  Inputs=3
  Mux1 : Mux  Inputs=2
  Mux2 : Mux  Inputs=2
  Product 1 : Product  Multiplication=Matrix(*)
  Right Angular Velocity3 : Scope
      settings: YMin=-1  YMax=1  SaveName=ScopeData30
  Sum2 : Sum  Inputs=|+-
  Sum4 : Sum  Inputs=+++
  Unit Delay 7 : UnitDelay  InitialCondition=[2500 200 0]'  SampleTime=-1
  X_i : Outport
  Theta_i : Outport  Port=2
  wires:
  Mux1/1 -> Fcn 2/1
  Delta_s,c/1 -> Mux1/1, Mux2/1
  Delta_theta,c/1 -> Mux/3
  Mux2/1 -> Fcn 1/1
  Fcn 1/1 -> Mux/1
  Fcn 2/1 -> Mux/2
  Sum4/1 -> X_i/1, Gain 1/1, Unit Delay 7/1, Gain 2/1, Right Angular Velocity3/1, Gain 6/1
  Gain 6/1 -> Mux1/2, Mux2/2
  Z_i/1 -> Sum2/1
  Gain 1/1 -> Sum2/2
  Sum2/1 -> Product 1/2
  K_i/1 -> Product 1/1
  Unit Delay 7/1 -> Sum4/1
  Mux/1 -> Sum4/2
  Product 1/1 -> Sum4/3
  Gain 2/1 -> Theta_i/1

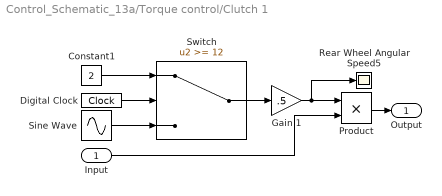
== system Control_Schematic_13a/Torque control/Clutch 1 ==
  Input : Inport
  Constant1 : Constant  Value=2
  Digital Clock : DigitalClock  SampleTime=Ts
  Gain 1 : Gain  Gain=.5
  Product : Product
  Rear Wheel Angular Speed5 : Scope
      settings: YMin=0  YMax=1  SaveName=ScopeData20
  Sine Wave : Sin  Bias=1  Frequency=(pi/12)  Phase=-pi/2  SampleTime=Ts
  Switch : Switch  Threshold=12
  Output : Outport
  wires:
  Constant1/1 -> Switch/1
  Digital Clock/1 -> Switch/2
  Switch/1 -> Gain 1/1
  Input/1 -> Product/2
  Product/1 -> Output/1
  Sine Wave/1 -> Switch/3
  Gain 1/1 -> Rear Wheel Angular Speed5/1, Product/1

== system Control_Schematic_13a/Torque control/Clutch 2 ==
  Input : Inport
  Constant1 : Constant  Value=2
  Digital Clock : DigitalClock  SampleTime=Ts
  Gain 1 : Gain  Gain=.5
  Product : Product
  Rear Wheel Angular Speed5 : Scope
      settings: YMin=0  YMax=1  SaveName=ScopeData20
  Sine Wave : Sin  Bias=1  Frequency=(pi/12)  Phase=-pi/2  SampleTime=Ts
  Switch : Switch  Threshold=12
  Output : Outport
  wires:
  Gain 1/1 -> Product/1, Rear Wheel Angular Speed5/1
  Sine Wave/1 -> Switch/3
  Product/1 -> Output/1
  Input/1 -> Product/2
  Switch/1 -> Gain 1/1
  Digital Clock/1 -> Switch/2
  Constant1/1 -> Switch/1

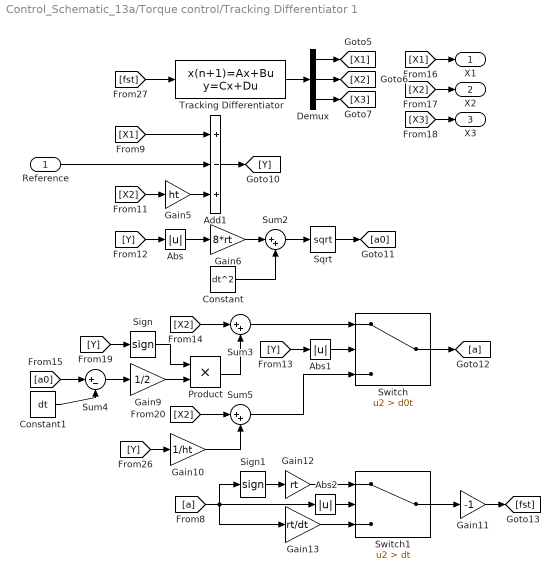
== system Control_Schematic_13a/Torque control/Tracking Differentiator 1 ==
  Reference : Inport
  Abs : Abs
  Abs1 : Abs
  Abs2 : Abs
  Add1 : Sum  Inputs=+-+
  Constant : Constant  Value=dt^2
  Constant1 : Constant  Value=dt
  Demux : Demux  Outputs=3
  Gain10 : Gain  Gain=1/ht
  Gain11 : Gain  Gain=-1
  Gain12 : Gain  Gain=rt
  Gain13 : Gain  Gain=rt/dt
  Gain5 : Gain  Gain=ht
  Gain6 : Gain  Gain=8*rt
  Gain9 : Gain  Gain=1/2
  Product : Product
  Sign : Signum
  Sign1 : Signum
  Sqrt : Sqrt  SaturateOnIntegerOverflow=on
  Sum2 : Sum  Inputs=|++
  Sum3 : Sum  Inputs=|++
  Sum4 : Sum  Inputs=|+-
  Sum5 : Sum  Inputs=|++
  Switch : Switch  Criteria=u2 > Threshold  Threshold=d0t
  Switch1 : Switch  Criteria=u2 > Threshold  Threshold=dt
  Tracking Differentiator : DiscreteStateSpace  A=TD.a  B=TD.b  C=TD.c  D=TD.d  SampleTime=Ts
  X1 : Outport
  X2 : Outport  Port=2
  X3 : Outport  Port=3
  wires:
  Gain11/1 -> [fst]
  Abs2/1 -> Switch1/2
  [Y] -> Gain10/1
  Sum5/1 -> Switch/3
  Switch/1 -> [a]
  [Y] -> Sign/1
  Switch1/1 -> Gain11/1
  [a] -> Abs2/1, Sign1/1, Gain13/1
  Gain10/1 -> Sum5/2
  [fst] -> Tracking Differentiator/1
  [X2] -> Sum5/1
  Constant1/1 -> Sum4/2
  Sign/1 -> Product/1
  Product/1 -> Sum3/2
  [a0] -> Sum4/1
  Gain13/1 -> Switch1/3
  Sum4/1 -> Gain9/1
  [X2] -> Sum3/1
  Sum3/1 -> Switch/1
  [Y] -> Abs1/1
  Gain9/1 -> Product/2
  Sign1/1 -> Gain12/1
  Abs1/1 -> Switch/2
  Sum2/1 -> Sqrt/1
  Sqrt/1 -> [a0]
  Constant/1 -> Sum2/2
  Abs/1 -> Gain6/1
  Gain6/1 -> Sum2/1
  [Y] -> Abs/1
  Demux/2 -> [X2]
  Tracking Differentiator/1 -> Demux/1
  Demux/3 -> [X3]
  Demux/1 -> [X1]
  Add1/1 -> [Y]
  [X1] -> X1/1
  Reference/1 -> Add1/2
  [X2] -> Gain5/1
  [X2] -> X2/1
  Gain12/1 -> Switch1/1
  [X1] -> Add1/1
  Gain5/1 -> Add1/3
  [X3] -> X3/1

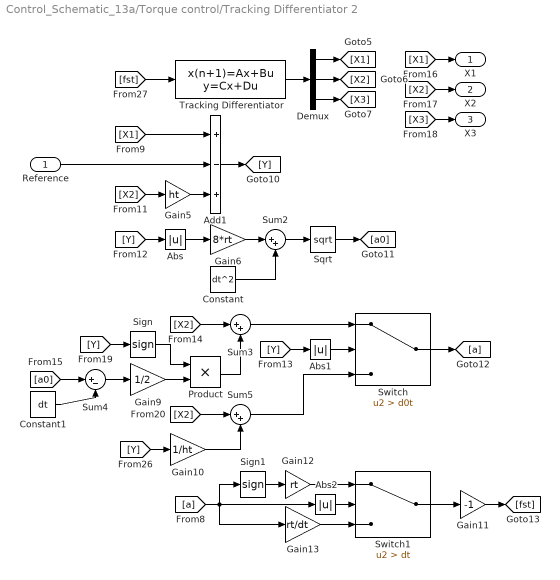
== system Control_Schematic_13a/Torque control/Tracking Differentiator 2 ==
  Reference : Inport
  Abs : Abs
  Abs1 : Abs
  Abs2 : Abs
  Add1 : Sum  Inputs=+-+
  Constant : Constant  Value=dt^2
  Constant1 : Constant  Value=dt
  Demux : Demux  Outputs=3
  Gain10 : Gain  Gain=1/ht
  Gain11 : Gain  Gain=-1
  Gain12 : Gain  Gain=rt
  Gain13 : Gain  Gain=rt/dt
  Gain5 : Gain  Gain=ht
  Gain6 : Gain  Gain=8*rt
  Gain9 : Gain  Gain=1/2
  Product : Product
  Sign : Signum
  Sign1 : Signum
  Sqrt : Sqrt  SaturateOnIntegerOverflow=on
  Sum2 : Sum  Inputs=|++
  Sum3 : Sum  Inputs=|++
  Sum4 : Sum  Inputs=|+-
  Sum5 : Sum  Inputs=|++
  Switch : Switch  Criteria=u2 > Threshold  Threshold=d0t
  Switch1 : Switch  Criteria=u2 > Threshold  Threshold=dt
  Tracking Differentiator : DiscreteStateSpace  A=TD.a  B=TD.b  C=TD.c  D=TD.d  SampleTime=Ts
  X1 : Outport
  X2 : Outport  Port=2
  X3 : Outport  Port=3
  wires:
  [X3] -> X3/1
  Gain5/1 -> Add1/3
  [X1] -> Add1/1
  Gain12/1 -> Switch1/1
  [X2] -> X2/1
  [X2] -> Gain5/1
  Reference/1 -> Add1/2
  [X1] -> X1/1
  Add1/1 -> [Y]
  Demux/1 -> [X1]
  Demux/3 -> [X3]
  Tracking Differentiator/1 -> Demux/1
  Demux/2 -> [X2]
  [Y] -> Abs/1
  Gain6/1 -> Sum2/1
  Abs/1 -> Gain6/1
  Constant/1 -> Sum2/2
  Sqrt/1 -> [a0]
  Sum2/1 -> Sqrt/1
  Abs1/1 -> Switch/2
  Sign1/1 -> Gain12/1
  Gain9/1 -> Product/2
  [Y] -> Abs1/1
  Sum3/1 -> Switch/1
  [X2] -> Sum3/1
  Sum4/1 -> Gain9/1
  Gain13/1 -> Switch1/3
  [a0] -> Sum4/1
  Product/1 -> Sum3/2
  Sign/1 -> Product/1
  Constant1/1 -> Sum4/2
  [X2] -> Sum5/1
  [fst] -> Tracking Differentiator/1
  Gain10/1 -> Sum5/2
  [a] -> Gain13/1, Sign1/1, Abs2/1
  Switch1/1 -> Gain11/1
  [Y] -> Sign/1
  Switch/1 -> [a]
  Sum5/1 -> Switch/3
  [Y] -> Gain10/1
  Abs2/1 -> Switch1/2
  Gain11/1 -> [fst]
